simulink model "peregrine_falcon_dive_part_2"  (R2024a)
settings: Solver=VariableStepAuto  StartTime=0.0  StopTime=2.5  RelTol=1e-3
StartFcn:
  | learning.simulink.modelCallbacks.startFunction(gcs)
StopFcn:
  | learning.simulink.modelCallbacks.stopFunction(gcs);
model workspace (MAT data in the model file):
  courseObject.course = 'simulink'
  courseObject.chapter = 13
  courseObject.lesson = 1
  courseObject.section = 3
  courseObject.task = 1
  t_ans = [0; 2.00950914521e-05; 0.000120570548712; 0.000622947835014; 0.00313483426652; 0.0156942664241; 0.0656942664241; 0.115694266424; 0.165694266424; 0.215694266424; 0.265694266424; 0.315694266424; 0.365694266424; 0.415694266424; 0.465694266424; 0.515694266424; 0.565694266424; 0.615694266424; 0.665694266424; 0.715694266424; 0.765694266424; 0.815694266424; 0.865694266424; 0.915694266424; 0.965694266424; 1.01569426642; 1.06569426642; 1.11569426642; 1.16569426642; 1.21569426642; 1.26569426642; 1.31569426642; 1.36569426642; 1.41569426642; 1.46569426642; 1.51569426642; 1.56569426642; 1.61569426642; 1.66569426642; 1.71569426642; 1.76569426642; 1.81569426642; 1.86569426642; 1.91569426642; 1.96569426642; 2.01569426642; 2.06569426642; 2.11569426642; 2.16569426642; 2.19463457714; 2.19463457714; 2.24463457714; 2.29463457714; 2.34463457714; 2.39463457714; 2.44463457714; 2.49463457714; 2.5]
  y_ans = [0; -0.00020095269191; -0.00120576947271; -0.00623118635213; -0.0313915881622; -0.158025658622; -0.811886886796; -1.92341395295; -3.11961857753; -4.39848606086; -5.75791544636; -7.19573192321; -8.70969910508; -10.2975310624; -11.9569039987; -13.6854674743; -15.4808550983; -17.3406946184; -19.26261736; -21.2442669734; -23.2833074637; -25.3774304913; -27.5243619387; -29.7218677519; -31.9677590705; -34.2598966706; -36.5961947476; -38.9746240733; -39.3623931929; -39.3623931929; -41.7872863785; -44.2501294833; -46.7490864731; -49.2823851453; -51.8483176758; -54.4452407868; -57.0715755761; -59.7258070456; -62.4064833651; -65.1122149071; -67.841673084; -70.5935890179; -73.3667520715; -76.1600082643; -78.9722585982; -81.8024573132; -84.6496100921; -87.5127722302; -90.3910467864; -93.2835827274; -96.1895730764; -99.1082530781; -102.038898385; -104.980823277; -107.933378914; -110.895951634; -113.867961291; -116.848859649; -119.838128823; -122.835279769; -125.839850838; -128.851406374; -131.869535374; -134.893850203; -137.923985356; -140.959596285; -144.000358268; -147.045965337; -150.096129253; -153.150578531; -156.209057513; -159.271325484; -162.337155837; -165.406335278; -168.478663068; -171.553950316; -174.632019295; -177.712702807; -180.795843571; -183.881293657; -186.968913936; -190.058573573; -193.150149544; -196.243526173; -199.338594709; -202.435252911; -205.533404672; -208.632959651; -211.733832935; -214.835944717; -217.93921999; -221.043588266; -224.148983305; -227.25534286; -230.362608441; -233.47072509; -236.579641166; -239.689308154; -242.799680468; -245.910715283; -249.022372364; -252.134613915; -255.247404426; -258.36071054; -261.474500922; -264.588746138; -267.703418537; -270.818492146; -270.98563988]
  y_ans2 = [60; 59.9997990471; 59.9987942238; 59.9937686328; 59.9686038259; 59.8418585583; 59.1851106103; 58.0601614461; 56.8381509288; 55.5192576032; 54.1036738006; 52.591605528; 50.9832723485; 49.2789072555; 47.4787565386; 45.5830796431; 43.5921490226; 41.506249984; 39.3256805272; 37.0507511771; 34.6817848108; 32.2191164776; 29.663093214; 27.0140738525; 24.2724288262; 21.4385399665; 18.512800298; 15.4956138266; 15; 15; 11.9211982055; 8.83982594906; 5.75603789236; 2.66997950169; -0.418212418155; -3.50840921969; -6.60048993647; -9.69434083345; -12.7898549826; -15.8869318625; -18.9854769806; -22.0854015173; -25.1866219898; -28.2890599361; -31.3926416164; -34.4972977326; -37.6029631632; -40.7095767147; -43.8170808864; -46.9254216501; -50.0345482416; -53.1444129656; -56.2549710112; -59.3661802789; -62.4780012174; -65.5903966704; -68.7033317326; -71.8167736137; -74.9306915113; -78.0450564906; -81.1598413719; -84.2750206244; -87.3905702669; -90.5064677736; -93.6226919866; -96.7392230326; -99.8560422456; -102.973132094; -106.090476109; -109.208058827; -112.325865721; -115.443883147; -118.562098293; -121.680499123; -124.799074335; -127.917813314; -131.03670609; -134.155743301; -137.274916152; -140.394216385; -143.513636245; -146.633168447; -149.752806151; -152.872542932; -155.992372757; -159.11228996; -162.23228922; -165.352365538; -168.472514224; -171.592730868; -174.713011332; -177.83335173; -180.95374841; -184.074197944; -187.194697114; -190.315242896; -193.435832451; -196.556463112; -199.677132376; -202.797837891; -205.91857745; -209.039348978; -212.160150527; -215.28098027; -218.401836489; -221.52271757; -224.643622; -227.764548356; -227.931999846]
  y_ans3 = [60; 59.9997990471; 59.9987942238; 59.9937686328; 59.9686038259; 59.8418585583; 59.3220582559; 58.7779462171; 58.2095423654; 57.616867496; 56.9999432736; 56.3587922284; 55.6934377533; 55.0039041004; 54.2902163776; 53.5524005447; 52.7904834099; 52.0044926258; 51.1944566854; 50.3604049183; 49.502367486; 48.6203753781; 47.7144604076; 46.7846552062; 45.83099322; 44.8535087047; 43.8522367205; 42.8272131275; 41.7784745802; 40.7060585227; 39.6100031835; 38.4903475698; 37.3471314624; 36.1803954098; 34.990180723; 33.7765294693; 32.539484467; 31.2790892792; 29.9953882076; 28.6884262869; 27.3582492785; 26.004903664; 24.6284366393; 23.2288961078; 21.8063306743; 20.3607896383; 18.8923229872; 17.4009813902; 15.8868161908; 15; 15; 13.4609304512; 11.9211982055; 10.3808234967; 8.83982594908; 7.29822459501; 5.75603789239; 5.5905141921]
undefined symbols (not defined in the file): A1, A2, Cd1, Cd2, g, m, rho
CloseFcn:
  | learning.simulink.cleanupOnlineTraining;learning.simulink.Application.getInstance().dduxLogMatlabEvent("ModelClosed")
Description:
  | TrainingCourseModel
settings Model: Creator=hp  LastModifiedBy=hp
settings DataIOCC: SaveTime=off
settings RTWCC: GPUComputeCapability=3.5

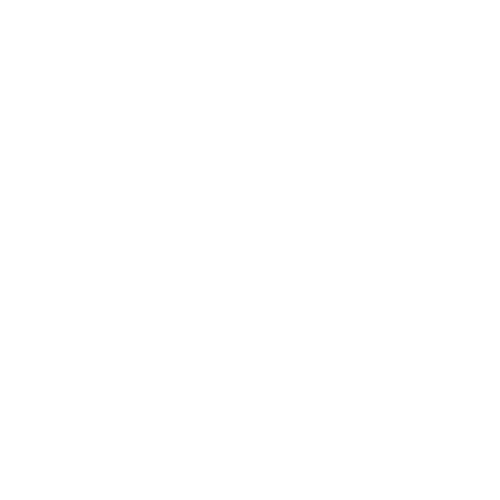
[thumbnail: Simulink's stored preview of the top-level diagram]
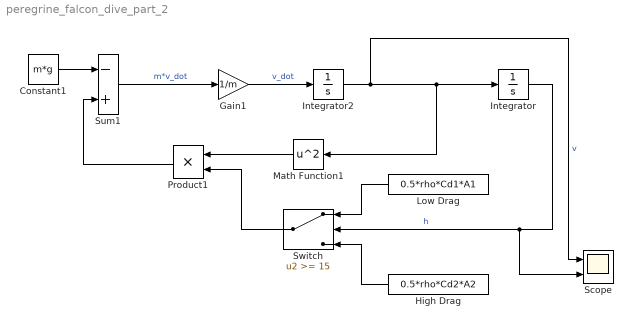
== system peregrine_falcon_dive_part_2 ==
  Constant1 : Constant  Value=m*g
  Gain1 : Gain  Gain=1/m
  High Drag : Constant  Value=0.5*rho*Cd2*A2
  Integrator : Integrator  InitialCondition=60
  Integrator2 : Integrator  InitialCondition=-10
  Low Drag : Constant  Value=0.5*rho*Cd1*A1
  Math Function1 : Math  Operator=square  SignedPower=on
  Product1 : Product
  Scope : Scope  NumInputPorts=2
  Sum1 : Sum  Inputs=-+
  Switch : Switch  Threshold=15  SaturateOnIntegerOverflow=off  InputSameDT=off
  wires:
  Constant1/1 -> Sum1/1
  Integrator2/1 -> Scope/1, Integrator/1, Math Function1/1  "v"
  Gain1/1 -> Integrator2/1  "v_dot"
  Product1/1 -> Sum1/2
  Sum1/1 -> Gain1/1  "m*v_dot"
  Math Function1/1 -> Product1/1
  Switch/1 -> Product1/2
  Low Drag/1 -> Switch/1
  High Drag/1 -> Switch/3
  Integrator/1 -> Scope/2, Switch/2  "h"
